simulink model "mohupid"  (R2022b)
settings: Solver=VariableStepAuto  StartTime=0.0  StopTime=3  FixedStep=0.01  RelTol=1e-5
libraries: slpidlib x4, fuzblock x3
settings Model: Creator=邹舸  LastModifiedBy=邹舸

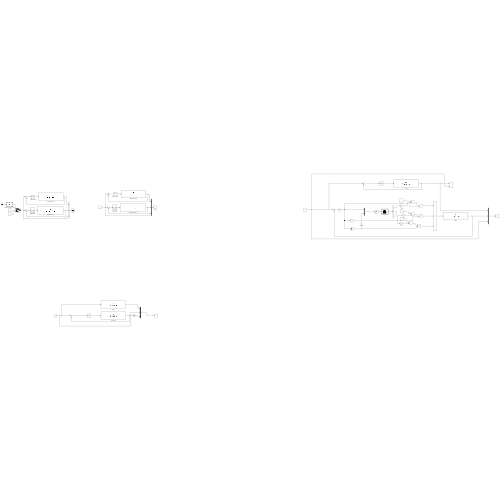
[thumbnail: Simulink's stored preview of the top-level diagram]
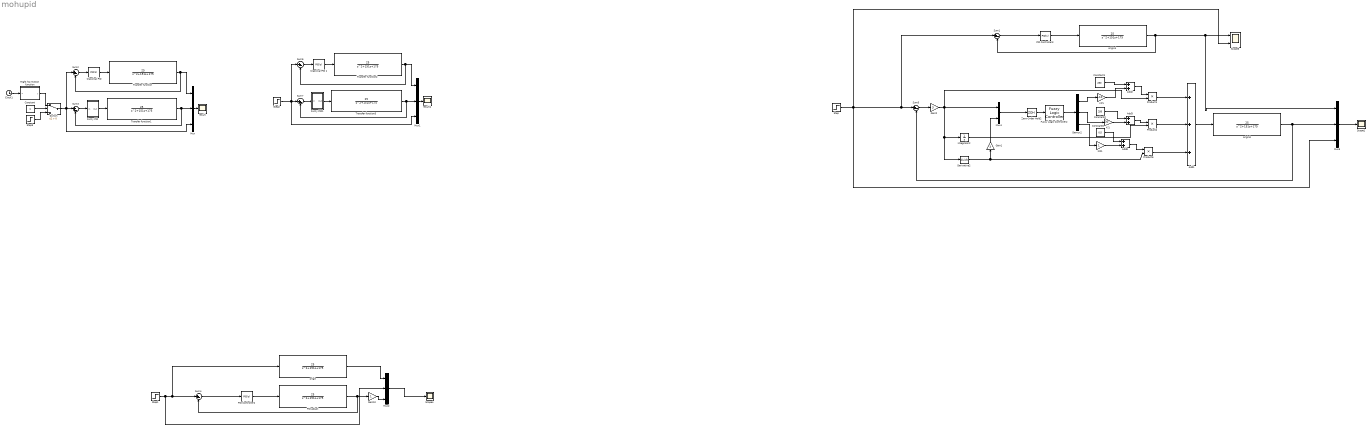
== system mohupid ==
  " Classical PID " : slpidlib/PID Controller  Controller=PID  Form=Parallel  TimeDomain=Continuous-time  UseExternalTs=off  SampleTime=-1  IntegratorMethod=Forward Euler  FilterMethod=Forward Euler  ControllerParametersSource=internal  P=450  I=250  UseKiTs=off  D=3  N=20.6893403846327  UseFilter=on  TunerSelectOption=Transfer Function Based (PID Tuner App)  InitialConditionSource=internal  InitialConditionForIntegrator=0  InitialConditionForFilter=0  DifferentiatorICPrevScaledInput=0  ExternalReset=none  TrackingMode=off  Kt=1  LimitOutput=off  SatLimitsSource=internal  UpperSaturationLimit=inf  LowerSaturationLimit=-inf  LinearizeAsGain=on  AntiWindupMode=none  Kb=1  LimitIntegrator=off  UpperIntegratorSaturationLimit=inf  LowerIntegratorSaturationLimit=-inf  POutMin=[]  POutMax=[]  IOutMin=[]  IOutMax=[]  DOutMin=[]  DOutMax=[]  NOutMin=[]  NOutMax=[]  SumOutMin=[]  SumOutMax=[]  SaturationOutMin=[]  SaturationOutMax=[]  PParamMin=[]  PParamMax=[]  IParamMin=[]  IParamMax=[]  DParamMin=[]  DParamMax=[]  NParamMin=[]  NParamMax=[]  KbParamMin=[]  KbParamMax=[]  KtParamMin=[]  KtParamMax=[]  KbOutMin=[]  KbOutMax=[]  KtOutMin=[]  KtOutMax=[]  IntegratorOutMin=[]  IntegratorOutMax=[]  FilterOutMin=[]  FilterOutMax=[]  SumI1OutMin=[]  SumI1OutMax=[]  SumI2OutMin=[]  SumI2OutMax=[]  SumI3OutMin=[]  SumI3OutMax=[]  SumI4OutMin=[]  SumI4OutMax=[]  SumDOutMin=[]  SumDOutMax=[]  DifferentiatorOutMin=[]  DifferentiatorOutMax=[]  FilterDiffOutCoefMin=[]  FilterDiffOutCoefMax=[]  ReciprocalOutMin=[]  ReciprocalOutMax=[]  SumDenOutMin=[]  SumDenOutMax=[]  SumNumOutMin=[]  SumNumOutMax=[]  DivideOutMin=[]  DivideOutMax=[]  UdiffTsProdOutMin=[]  UdiffTsProdOutMax=[]  NTsProdOutMin=[]  NTsProdOutMax=[]  UintegralTsProdOutMin=[]  UintegralTsProdOutMax=[]  UngainTsProdOutMin=[]  UngainTsProdOutMax=[]  ClampingZeroOutDataTypeStr=Inherit: Inherit via back propagation  ClampingZeroOutMin=[]  ClampingZeroOutMax=[]  FilterDenConstantOutDataTypeStr=Inherit: Inherit via back propagation  FilterDenConstantOutMin=[]  FilterDenConstantOutMax=[]  PCopyOutDataTypeStr=Inherit: Inherit via back propagation  PCopyOutMin=[]  PCopyOutMax=[]  NCopyOutDataTypeStr=Inherit: Inherit via back propagation  NCopyOutMin=[]  NCopyOutMax=[]  IntegratorContinuousStateAttributes=''  IntegratorStateMustResolveToSignalObject=off  IntegratorRTWStateStorageClass=Auto  FilterContinuousStateAttributes=''  FilterStateMustResolveToSignalObject=off  FilterRTWStateStorageClass=Auto  ParallelPVariant=InternalParameters  IdealPVariant=Disabled  IVariant=InternalParameters  DVariant=InternalParameters  IntegratorVariant=Continuous  SatVariant=Disabled  AWVariant=Passthrough  PCopyVariant=Disabled  TRVariant=Disabled  FdbkBlocksVariant=Forward  IdealPFdbkVariant=Disabled  SatFdbkVariant=Disabled  DerivativeFilterVariant=ContFilter  NVariant=InternalParameters  NCopyVariant=Disabled  FilterICVariant=InternalICsFilter  IntegratorICVariant=InternalICs  ExternalResetVariant=Disabled  TRSumVariant=Passthrough  SumFdbkVariant=Disabled  SumVariant=Sum_PID  TsampFilterVariant=InternalTs  TsampNgainVariant=Passthrough  TsampIntegralVariant=Passthrough  ExternalSaturationOutDataTypeStr=Inherit: Same as second input
  " Classical PID 1" : slpidlib/PID Controller  Controller=PID  Form=Parallel  TimeDomain=Continuous-time  UseExternalTs=off  SampleTime=-1  IntegratorMethod=Forward Euler  FilterMethod=Forward Euler  ControllerParametersSource=internal  P=450  I=200  UseKiTs=off  D=3  N=20.6893403846327  UseFilter=on  TunerSelectOption=Transfer Function Based (PID Tuner App)  InitialConditionSource=internal  InitialConditionForIntegrator=0  InitialConditionForFilter=0  DifferentiatorICPrevScaledInput=0  ExternalReset=none  TrackingMode=off  Kt=1  LimitOutput=off  SatLimitsSource=internal  UpperSaturationLimit=inf  LowerSaturationLimit=-inf  LinearizeAsGain=on  AntiWindupMode=none  Kb=1  LimitIntegrator=off  UpperIntegratorSaturationLimit=inf  LowerIntegratorSaturationLimit=-inf  POutMin=[]  POutMax=[]  IOutMin=[]  IOutMax=[]  DOutMin=[]  DOutMax=[]  NOutMin=[]  NOutMax=[]  SumOutMin=[]  SumOutMax=[]  SaturationOutMin=[]  SaturationOutMax=[]  PParamMin=[]  PParamMax=[]  IParamMin=[]  IParamMax=[]  DParamMin=[]  DParamMax=[]  NParamMin=[]  NParamMax=[]  KbParamMin=[]  KbParamMax=[]  KtParamMin=[]  KtParamMax=[]  KbOutMin=[]  KbOutMax=[]  KtOutMin=[]  KtOutMax=[]  IntegratorOutMin=[]  IntegratorOutMax=[]  FilterOutMin=[]  FilterOutMax=[]  SumI1OutMin=[]  SumI1OutMax=[]  SumI2OutMin=[]  SumI2OutMax=[]  SumI3OutMin=[]  SumI3OutMax=[]  SumI4OutMin=[]  SumI4OutMax=[]  SumDOutMin=[]  SumDOutMax=[]  DifferentiatorOutMin=[]  DifferentiatorOutMax=[]  FilterDiffOutCoefMin=[]  FilterDiffOutCoefMax=[]  ReciprocalOutMin=[]  ReciprocalOutMax=[]  SumDenOutMin=[]  SumDenOutMax=[]  SumNumOutMin=[]  SumNumOutMax=[]  DivideOutMin=[]  DivideOutMax=[]  UdiffTsProdOutMin=[]  UdiffTsProdOutMax=[]  NTsProdOutMin=[]  NTsProdOutMax=[]  UintegralTsProdOutMin=[]  UintegralTsProdOutMax=[]  UngainTsProdOutMin=[]  UngainTsProdOutMax=[]  ClampingZeroOutDataTypeStr=Inherit: Inherit via back propagation  ClampingZeroOutMin=[]  ClampingZeroOutMax=[]  FilterDenConstantOutDataTypeStr=Inherit: Inherit via back propagation  FilterDenConstantOutMin=[]  FilterDenConstantOutMax=[]  PCopyOutDataTypeStr=Inherit: Inherit via back propagation  PCopyOutMin=[]  PCopyOutMax=[]  NCopyOutDataTypeStr=Inherit: Inherit via back propagation  NCopyOutMin=[]  NCopyOutMax=[]  IntegratorContinuousStateAttributes=''  IntegratorStateMustResolveToSignalObject=off  IntegratorRTWStateStorageClass=Auto  FilterContinuousStateAttributes=''  FilterStateMustResolveToSignalObject=off  FilterRTWStateStorageClass=Auto  ParallelPVariant=InternalParameters  IdealPVariant=Disabled  IVariant=InternalParameters  DVariant=InternalParameters  IntegratorVariant=Continuous  SatVariant=Disabled  AWVariant=Passthrough  PCopyVariant=Disabled  TRVariant=Disabled  FdbkBlocksVariant=Forward  IdealPFdbkVariant=Disabled  SatFdbkVariant=Disabled  DerivativeFilterVariant=ContFilter  NVariant=InternalParameters  NCopyVariant=Disabled  FilterICVariant=InternalICsFilter  IntegratorICVariant=InternalICs  ExternalResetVariant=Disabled  TRSumVariant=Passthrough  SumFdbkVariant=Disabled  SumVariant=Sum_PID  TsampFilterVariant=InternalTs  TsampNgainVariant=Passthrough  TsampIntegralVariant=Passthrough  ExternalSaturationOutDataTypeStr=Inherit: Same as second input
  Add1 : Sum  Inputs=+++
  Add2 : Sum
  Add3 : Sum
  Add8 : Sum
  Clock1 : Clock
      settings: Decimation=4
  Constant : Constant
  Constant1 : Constant  Value=250
  Constant2 : Constant  Value=250
  Constant6 : Constant  Value=0.5
  Demux2 : Demux  Outputs=3
  Derivative2 : Derivative
  Fuzzy Logic Controller2 : fuzblock/Fuzzy Logic  Controller  FIS='rules.fis'  OutputSampleNumber=101  DataType=double  FuzzifiedInputs=off  RuleFiringStrengths=off  RuleOutputs=off  AggregatedOutputs=off  SimulateUsing=Interpreted execution  OutOfRangeInputValueMessage=warning  NoRuleFiredMessage=warning  EmptyOutputFuzzySetMessage=warning
  Fuzzy PID : Subsystem
  Fuzzy PID1 : Subsystem
  Gain1 : Gain  Gain=3
  Gain10 : Gain
  Gain2 : Gain  Gain=3
  Integrator2 : Integrator
  KD1 : Gain
  KI1 : Gain  Gain=30
  KP1 : Gain  Gain=-10
  Mux{,1..3} (4 alike) : Mux  Inputs=3
  Mux4 : Mux  Inputs=2
  PID Controller2 : slpidlib/PID Controller  Controller=PID  Form=Parallel  TimeDomain=Continuous-time  UseExternalTs=off  SampleTime=-1  IntegratorMethod=Forward Euler  FilterMethod=Forward Euler  ControllerParametersSource=internal  P=71.0435672102917  I=249.379351311442  UseKiTs=off  D=-0.543268347366237  N=130.770672642186  UseFilter=on  TunerSelectOption=Transfer Function Based (PID Tuner App)  InitialConditionSource=internal  InitialConditionForIntegrator=0  InitialConditionForFilter=0  DifferentiatorICPrevScaledInput=0  ExternalReset=none  TrackingMode=off  Kt=1  LimitOutput=off  SatLimitsSource=internal  UpperSaturationLimit=inf  LowerSaturationLimit=-inf  LinearizeAsGain=on  AntiWindupMode=none  Kb=1  LimitIntegrator=off  UpperIntegratorSaturationLimit=inf  LowerIntegratorSaturationLimit=-inf  POutMin=[]  POutMax=[]  IOutMin=[]  IOutMax=[]  DOutMin=[]  DOutMax=[]  NOutMin=[]  NOutMax=[]  SumOutMin=[]  SumOutMax=[]  SaturationOutMin=[]  SaturationOutMax=[]  PParamMin=[]  PParamMax=[]  IParamMin=[]  IParamMax=[]  DParamMin=[]  DParamMax=[]  NParamMin=[]  NParamMax=[]  KbParamMin=[]  KbParamMax=[]  KtParamMin=[]  KtParamMax=[]  KbOutMin=[]  KbOutMax=[]  KtOutMin=[]  KtOutMax=[]  IntegratorOutMin=[]  IntegratorOutMax=[]  FilterOutMin=[]  FilterOutMax=[]  SumI1OutMin=[]  SumI1OutMax=[]  SumI2OutMin=[]  SumI2OutMax=[]  SumI3OutMin=[]  SumI3OutMax=[]  SumI4OutMin=[]  SumI4OutMax=[]  SumDOutMin=[]  SumDOutMax=[]  DifferentiatorOutMin=[]  DifferentiatorOutMax=[]  FilterDiffOutCoefMin=[]  FilterDiffOutCoefMax=[]  ReciprocalOutMin=[]  ReciprocalOutMax=[]  SumDenOutMin=[]  SumDenOutMax=[]  SumNumOutMin=[]  SumNumOutMax=[]  DivideOutMin=[]  DivideOutMax=[]  UdiffTsProdOutMin=[]  UdiffTsProdOutMax=[]  NTsProdOutMin=[]  NTsProdOutMax=[]  UintegralTsProdOutMin=[]  UintegralTsProdOutMax=[]  UngainTsProdOutMin=[]  UngainTsProdOutMax=[]  ClampingZeroOutDataTypeStr=Inherit: Inherit via back propagation  ClampingZeroOutMin=[]  ClampingZeroOutMax=[]  FilterDenConstantOutDataTypeStr=Inherit: Inherit via back propagation  FilterDenConstantOutMin=[]  FilterDenConstantOutMax=[]  PCopyOutDataTypeStr=Inherit: Inherit via back propagation  PCopyOutMin=[]  PCopyOutMax=[]  NCopyOutDataTypeStr=Inherit: Inherit via back propagation  NCopyOutMin=[]  NCopyOutMax=[]  IntegratorContinuousStateAttributes=''  IntegratorStateMustResolveToSignalObject=off  IntegratorRTWStateStorageClass=Auto  FilterContinuousStateAttributes=''  FilterStateMustResolveToSignalObject=off  FilterRTWStateStorageClass=Auto  ParallelPVariant=InternalParameters  IdealPVariant=Disabled  IVariant=InternalParameters  DVariant=InternalParameters  IntegratorVariant=Continuous  SatVariant=Disabled  AWVariant=Passthrough  PCopyVariant=Disabled  TRVariant=Disabled  FdbkBlocksVariant=Forward  IdealPFdbkVariant=Disabled  SatFdbkVariant=Disabled  DerivativeFilterVariant=ContFilter  NVariant=InternalParameters  NCopyVariant=Disabled  FilterICVariant=InternalICsFilter  IntegratorICVariant=InternalICs  ExternalResetVariant=Disabled  TRSumVariant=Passthrough  SumFdbkVariant=Disabled  SumVariant=Sum_PID  TsampFilterVariant=InternalTs  TsampNgainVariant=Passthrough  TsampIntegralVariant=Passthrough  ExternalSaturationOutDataTypeStr=Inherit: Same as second input
  PID Controller3 : slpidlib/PID Controller  Controller=PID  Form=Parallel  TimeDomain=Continuous-time  UseExternalTs=off  SampleTime=-1  IntegratorMethod=Forward Euler  FilterMethod=Forward Euler  ControllerParametersSource=internal  P=250  I=250  UseKiTs=off  D=0.5  N=20.6893403846327  UseFilter=on  TunerSelectOption=Transfer Function Based (PID Tuner App)  InitialConditionSource=internal  InitialConditionForIntegrator=0  InitialConditionForFilter=0  DifferentiatorICPrevScaledInput=0  ExternalReset=none  TrackingMode=off  Kt=1  LimitOutput=off  SatLimitsSource=internal  UpperSaturationLimit=inf  LowerSaturationLimit=-inf  LinearizeAsGain=on  AntiWindupMode=none  Kb=1  LimitIntegrator=off  UpperIntegratorSaturationLimit=inf  LowerIntegratorSaturationLimit=-inf  POutMin=[]  POutMax=[]  IOutMin=[]  IOutMax=[]  DOutMin=[]  DOutMax=[]  NOutMin=[]  NOutMax=[]  SumOutMin=[]  SumOutMax=[]  SaturationOutMin=[]  SaturationOutMax=[]  PParamMin=[]  PParamMax=[]  IParamMin=[]  IParamMax=[]  DParamMin=[]  DParamMax=[]  NParamMin=[]  NParamMax=[]  KbParamMin=[]  KbParamMax=[]  KtParamMin=[]  KtParamMax=[]  KbOutMin=[]  KbOutMax=[]  KtOutMin=[]  KtOutMax=[]  IntegratorOutMin=[]  IntegratorOutMax=[]  FilterOutMin=[]  FilterOutMax=[]  SumI1OutMin=[]  SumI1OutMax=[]  SumI2OutMin=[]  SumI2OutMax=[]  SumI3OutMin=[]  SumI3OutMax=[]  SumI4OutMin=[]  SumI4OutMax=[]  SumDOutMin=[]  SumDOutMax=[]  DifferentiatorOutMin=[]  DifferentiatorOutMax=[]  FilterDiffOutCoefMin=[]  FilterDiffOutCoefMax=[]  ReciprocalOutMin=[]  ReciprocalOutMax=[]  SumDenOutMin=[]  SumDenOutMax=[]  SumNumOutMin=[]  SumNumOutMax=[]  DivideOutMin=[]  DivideOutMax=[]  UdiffTsProdOutMin=[]  UdiffTsProdOutMax=[]  NTsProdOutMin=[]  NTsProdOutMax=[]  UintegralTsProdOutMin=[]  UintegralTsProdOutMax=[]  UngainTsProdOutMin=[]  UngainTsProdOutMax=[]  ClampingZeroOutDataTypeStr=Inherit: Inherit via back propagation  ClampingZeroOutMin=[]  ClampingZeroOutMax=[]  FilterDenConstantOutDataTypeStr=Inherit: Inherit via back propagation  FilterDenConstantOutMin=[]  FilterDenConstantOutMax=[]  PCopyOutDataTypeStr=Inherit: Inherit via back propagation  PCopyOutMin=[]  PCopyOutMax=[]  NCopyOutDataTypeStr=Inherit: Inherit via back propagation  NCopyOutMin=[]  NCopyOutMax=[]  IntegratorContinuousStateAttributes=''  IntegratorStateMustResolveToSignalObject=off  IntegratorRTWStateStorageClass=Auto  FilterContinuousStateAttributes=''  FilterStateMustResolveToSignalObject=off  FilterRTWStateStorageClass=Auto  ParallelPVariant=InternalParameters  IdealPVariant=Disabled  IVariant=InternalParameters  DVariant=InternalParameters  IntegratorVariant=Continuous  SatVariant=Disabled  AWVariant=Passthrough  PCopyVariant=Disabled  TRVariant=Disabled  FdbkBlocksVariant=Forward  IdealPFdbkVariant=Disabled  SatFdbkVariant=Disabled  DerivativeFilterVariant=ContFilter  NVariant=InternalParameters  NCopyVariant=Disabled  FilterICVariant=InternalICsFilter  IntegratorICVariant=InternalICs  ExternalResetVariant=Disabled  TRSumVariant=Passthrough  SumFdbkVariant=Disabled  SumVariant=Sum_PID  TsampFilterVariant=InternalTs  TsampNgainVariant=Passthrough  TsampIntegralVariant=Passthrough  ExternalSaturationOutDataTypeStr=Inherit: Same as second input
  PID adjust : TransferFcn  Numerator=[25]  Denominator=[1 151 175]
  Product1 : Product
  Product2 : Product
  Product6 : Product
  Right hip motion function : MATLAB Function  TreatAsAtomicUnit=on
  Scope1 : Scope
  Scope3 : Scope  NumInputPorts=2
  Scope4 : Scope
  Step{,1..3} (4 alike) : Step  Time=0  SampleTime=0
  Sum{1..7} (7 alike) : Sum  Inputs=|+-
  Switch : Switch  Criteria=u2 > Threshold  SaturateOnIntegerOverflow=off  InputSameDT=off
  Transfer function{,1..3} (4 alike) : TransferFcn  Numerator=[25]  Denominator=[1 151 175]
  Zero-Order Hold2 : ZeroOrderHold  SampleTime=-1
  origin : TransferFcn  Numerator=[25]  Denominator=[1 151 175]
  origin3 : TransferFcn  Numerator=[25]  Denominator=[1 151 175]
  origin4 : TransferFcn  Numerator=[25]  Denominator=[1 151 175]
  result : Scope
  result1 : Scope
  wires:
  Sum2/1 -> " Classical PID "/1
  Transfer function/1 -> Sum2/2, Mux/1
  " Classical PID "/1 -> Transfer function/1
  PID Controller2/1 -> PID adjust/1
  PID adjust/1 -> Gain10/1, Sum4/2
  Sum4/1 -> PID Controller2/1
  Step1/1 -> Mux2/2, origin/1, Sum4/1
  Mux2/1 -> Scope4/1
  origin/1 -> Mux2/1
  Gain10/1 -> Mux2/3
  Clock1/1 -> Right hip motion function/1(u)
  Transfer function1/1 -> Mux/2, Sum3/2
  Mux/1 -> result/1
  Mux3/1 -> Scope1/1
  origin3/1 -> Mux3/2, Sum5/2
  Gain1/1 -> Mux4/2
  PID Controller3/1 -> origin4/1
  origin4/1 -> Mux3/1, Scope3/1, Sum1/2
  Sum1/1 -> PID Controller3/1
  Step/1 -> Mux3/3, Sum1/1, Sum5/1, Scope3/2
  Sum5/1 -> Gain2/1
  Derivative2/1 -> Gain1/1, Product6/2
  Integrator2/1 -> Product2/2
  Constant1/1 -> Add2/1
  Add2/1 -> Product1/1
  Constant2/1 -> Add3/1
  Constant6/1 -> Add8/1
  Add3/1 -> Product2/1
  Add8/1 -> Product6/1
  Demux2/1 -> KP1/1
  Demux2/2 -> KI1/1
  Demux2/3 -> KD1/1
  Fuzzy Logic Controller2/1 -> Demux2/1
  Zero-Order Hold2/1 -> Fuzzy Logic Controller2/1
  Mux4/1 -> Zero-Order Hold2/1
  Product1/1 -> Add1/1
  Product2/1 -> Add1/2
  Product6/1 -> Add1/3
  Gain2/1 -> Integrator2/1, Derivative2/1, Product1/2, Mux4/1
  KP1/1 -> Add2/2
  KI1/1 -> Add3/2
  KD1/1 -> Add8/2
  Add1/1 -> origin3/1
  Sum3/1 -> Fuzzy PID/1(in)
  Fuzzy PID/1(Out) -> Transfer function1/1
  Fuzzy PID1/1(Out) -> Transfer function3/1
  Sum7/1 -> Fuzzy PID1/1(in)
  Mux1/1 -> result1/1
  Transfer function3/1 -> Sum7/2, Mux1/2
  " Classical PID 1"/1 -> Transfer function2/1
  Transfer function2/1 -> Mux1/1, Sum6/2
  Sum6/1 -> " Classical PID 1"/1
  Step2/1 -> Sum7/1, Mux1/3, Sum6/1
  Switch/1 -> Mux/3, Sum2/1, Sum3/1
  Step3/1 -> Switch/3
  Right hip motion function/1(y) -> Switch/1
  Constant/1 -> Switch/2

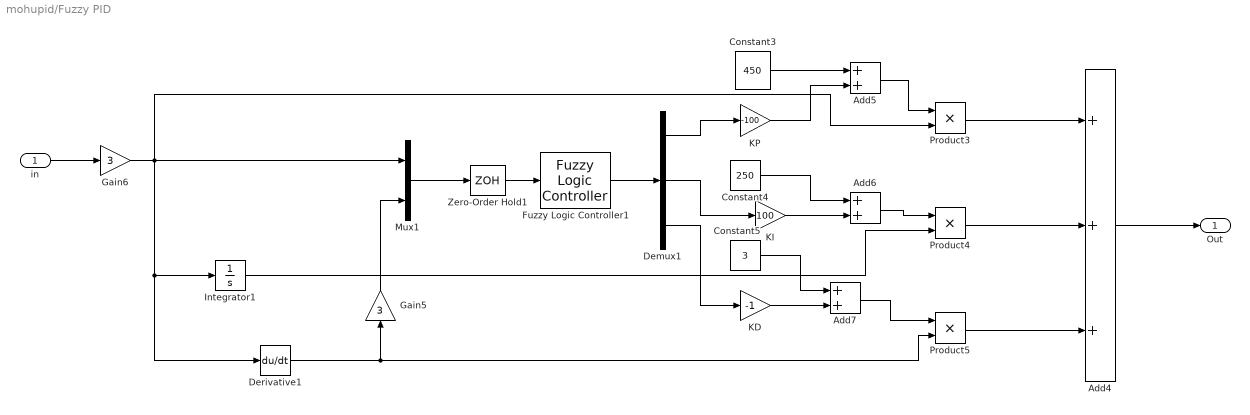
== system mohupid/Fuzzy PID ==
  in : Inport
  Add4 : Sum  Inputs=+++
  Add5 : Sum
  Add6 : Sum
  Add7 : Sum
  Constant3 : Constant  Value=450
  Constant4 : Constant  Value=250
  Constant5 : Constant  Value=3
  Demux1 : Demux  Outputs=3
  Derivative1 : Derivative
  Fuzzy Logic Controller1 : fuzblock/Fuzzy Logic  Controller  FIS='rules.fis'  OutputSampleNumber=101  DataType=double  FuzzifiedInputs=off  RuleFiringStrengths=off  RuleOutputs=off  AggregatedOutputs=off  SimulateUsing=Interpreted execution  OutOfRangeInputValueMessage=warning  NoRuleFiredMessage=warning  EmptyOutputFuzzySetMessage=warning
  Gain5 : Gain  Gain=3
  Gain6 : Gain  Gain=3
  Integrator1 : Integrator
  KD : Gain  Gain=-1
  KI : Gain  Gain=100
  KP : Gain  Gain=-100
  Mux1 : Mux  Inputs=2
  Product3 : Product
  Product4 : Product
  Product5 : Product
  Zero-Order Hold1 : ZeroOrderHold  SampleTime=-1
  Out : Outport
  wires:
  Gain6/1 -> Mux1/1, Product3/2, Derivative1/1, Integrator1/1
  Constant5/1 -> Add7/1
  Product5/1 -> Add4/3
  Demux1/1 -> KP/1
  Constant3/1 -> Add5/1
  Constant4/1 -> Add6/1
  KP/1 -> Add5/2
  Demux1/3 -> KD/1
  Derivative1/1 -> Gain5/1, Product5/2
  KD/1 -> Add7/2
  Zero-Order Hold1/1 -> Fuzzy Logic Controller1/1
  in/1 -> Gain6/1
  Add5/1 -> Product3/1
  Add7/1 -> Product5/1
  KI/1 -> Add6/2
  Gain5/1 -> Mux1/2
  Mux1/1 -> Zero-Order Hold1/1
  Product3/1 -> Add4/1
  Add6/1 -> Product4/1
  Integrator1/1 -> Product4/2
  Demux1/2 -> KI/1
  Fuzzy Logic Controller1/1 -> Demux1/1
  Product4/1 -> Add4/2
  Add4/1 -> Out/1

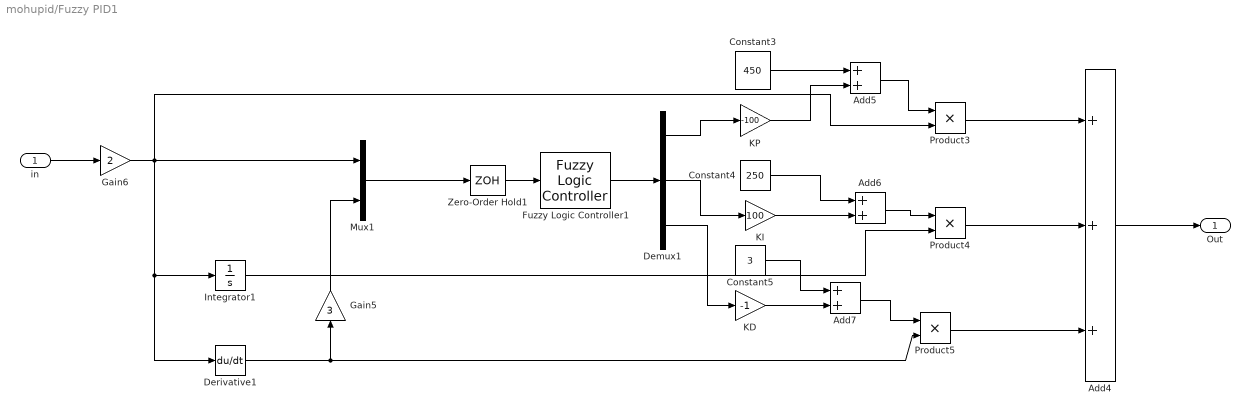
== system mohupid/Fuzzy PID1 ==
  in : Inport
  Add4 : Sum  Inputs=+++
  Add5 : Sum
  Add6 : Sum
  Add7 : Sum
  Constant3 : Constant  Value=450
  Constant4 : Constant  Value=250
  Constant5 : Constant  Value=3
  Demux1 : Demux  Outputs=3
  Derivative1 : Derivative
  Fuzzy Logic Controller1 : fuzblock/Fuzzy Logic  Controller  FIS='rules.fis'  OutputSampleNumber=101  DataType=double  FuzzifiedInputs=off  RuleFiringStrengths=off  RuleOutputs=off  AggregatedOutputs=off  SimulateUsing=Interpreted execution  OutOfRangeInputValueMessage=warning  NoRuleFiredMessage=warning  EmptyOutputFuzzySetMessage=warning
  Gain5 : Gain  Gain=3
  Gain6 : Gain  Gain=2
  Integrator1 : Integrator
  KD : Gain  Gain=-1
  KI : Gain  Gain=100
  KP : Gain  Gain=-100
  Mux1 : Mux  Inputs=2
  Product3 : Product
  Product4 : Product
  Product5 : Product
  Zero-Order Hold1 : ZeroOrderHold  SampleTime=-1
  Out : Outport
  wires:
  Add4/1 -> Out/1
  Product4/1 -> Add4/2
  Fuzzy Logic Controller1/1 -> Demux1/1
  Demux1/2 -> KI/1
  Integrator1/1 -> Product4/2
  Add6/1 -> Product4/1
  Product3/1 -> Add4/1
  Mux1/1 -> Zero-Order Hold1/1
  Gain5/1 -> Mux1/2
  KI/1 -> Add6/2
  Add7/1 -> Product5/1
  Add5/1 -> Product3/1
  in/1 -> Gain6/1
  Zero-Order Hold1/1 -> Fuzzy Logic Controller1/1
  KD/1 -> Add7/2
  Derivative1/1 -> Gain5/1, Product5/2
  Demux1/3 -> KD/1
  KP/1 -> Add5/2
  Constant4/1 -> Add6/1
  Constant3/1 -> Add5/1
  Demux1/1 -> KP/1
  Product5/1 -> Add4/3
  Constant5/1 -> Add7/1
  Gain6/1 -> Integrator1/1, Derivative1/1, Product3/2, Mux1/1

== matlab function mohupid/Right hip motion function ==
  data: u input; y output
function y = fcn(u)

y = 20.26*sin(5.126*u-1.436) +(-0.6631)*sin(6.249*u+-1.473) + 0.814*sin(4.749*u+-2.342) +  14.17*sin(0.005024*u+-0.1431) ...
+ 4.445*sin(10.24*u+4.138);
%-3.079+-0.2911*cos(u*1.651)+-0.9948*sin(u*1.651)
%          +-1.576*cos(2u*1.651)+-0.9949*sin(u*1.651)
%          +-3.536*cos(3u*1.651)+-0.9949*sin(u*1.651)
%          +0.2471*cos(4u*1.651)+-0.9949*sin(u*1.651)
%          +0.794*cos(5u*1.651)+-0.9949*sin(u*1.651)
%          +0.8891*cos(6u*1.651)+-0.9949*sin(u*1.651)
%          +-0.7193*cos(7u*1.651)+-0.9949*sin(u*1.651)
%          +0.5661*cos(8u*1.651)+-0.9949*sin(u*1.651)
